simulink library "simeventsserver1"  (Simulink 7.5)
settings: Solver=ode45  SolverMode=SingleTasking  StartTime=0.0  StopTime=10.0  RelTol=1e-3
undefined symbols (not defined in the file or in its folder): des_support, gcbh
settings Model: Creator=mclune  LastModifiedBy=ywu  ExtModeAutoUpdateStatusClock=off

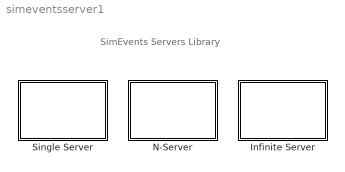
== system simeventsserver1 ==
  note: SimEvents Servers Library
  Infinite Server : Subsystem  Priority=1  LoadFcn=des_support('desLoadFcn',gcbh)  StartFcn=des_support('desStartFcn',gcbh)  StopFcn=des_support('desStopFcn',gcbh)  mask(Infinite Server){ServiceTimeFrom=Dialog, ServiceTime=1, AttributeName=ServiceTime, PriorityServiceCompletion=500, EnableTOPort=off, StatNumberDeparted=Off, StatNumberInBlock=Off, StatPendingEntity=Off, StatNumberPending=Off, StatAverageWait=Off, StatNumberTimedout=Off}
      mask prompts: ServiceTimeFrom "Service time from:"; ServiceTime "Service time:"; AttributeName "Attribute name:"; PriorityServiceCompletion "Service completion event priority:"; EnableTOPort "Enable TO port for timed-out entities:"; StatNumberDeparted "Number of entities departed, #d:"; StatNumberInBlock "Number of entities in block, #n:"; StatPendingEntity "Pending entity present in block, pe:"; StatNumberPending "Number of  pending entities, #pe:"; StatAverageWait "Average wait, w:"; StatNumberTimedout "Number of entities timed-out, #to:"
      mask help:
      | Delay any number of entities for a period of time and then attempt to output through the OUT port. If the OUT port is blocked then the entities stay in this block until the port becomes unblocked. You can specify the delay time via a parameter, attribute, or signal.
      | This block is an infinite server so the IN port is always available.
      mask init:
      | des_delaymask(gcb, 'init','apply')
      settings: CopyFcn=des_support('desCopyFcn',gcbh)  DeleteFcn=des_support('desDeleteFcn',gcbh)  UndoDeleteFcn=des_support('desUndoDeleteFcn',gcbh)  ModelCloseFcn=des_support('desModelCloseFcn',gcbh)  PreSaveFcn=des_support('desPreSaveFcn',gcbh)  PostSaveFcn=des_support('desPostSaveFcn',gcbh)  NameChangeFcn=des_support('desNameChangeFcn',gcbh)  CloseFcn=des_support('desCloseFcn',gcbh)  ErrorFcn=des_error_redirect
      mask Help: helpview(simeventsbhelp)
      mask StyleString: popup(Dialog|Signal port t|Attribute),edit,edit,edit,checkbox,popup(Off|On|Upon stop or pause),popup(Off|On|Upon stop or pause),popup(Off|On),popup(Off|On|Upon stop or pause),popup(Off|On|Upon stop or pause),popup(Off|On|Upon stop or pause)
      mask CallbackString: des_delaymask(gcb,'cbServiceTimeFrom','noapply');||||des_delaymask(gcb,'cbEnableTOPort','noapply');|des_delaymask(gcb,'cbStatNumberDeparted','noapply');|des_delaymask(gcb,'cbStatNumberInBlock','noapply');|des_delaymask(gcb,'cbStatPendingEntity','noapply');|des_delaymask(gcb,'cbStatNumberPending','noapply');|des_delaymask(gcb,'cbStatAverageWait','noapply');|des_delaymask(gcb,'cbStatNumberTimedout','noapply');
      mask TabNameString: Infinite Server,Infinite Server,Infinite Server,Infinite Server,Timeout,Statistics,Statistics,Statistics,Statistics,Statistics,Statistics
      mask Display:
      | image(des_iconLoad('serverInf.jpg'),'center');
      | port_label('LConn',1,'IN');
      | port_label('RConn',1,'OUT');
  N-Server : Subsystem  Priority=1  LoadFcn=des_support('desLoadFcn',gcbh)  StartFcn=des_support('desStartFcn',gcbh)  StopFcn=des_support('desStopFcn',gcbh)  mask(N-Server){NumberOfServers=5, ServiceTimeFrom=Dialog, ServiceTime=1, AttributeName=ServiceTime, PriorityServiceCompletion=500, EnableTOPort=off, StatNumberDeparted=Off, StatNumberInBlock=Off, StatPendingEntity=Off, StatNumberPending=Off, StatAverageWait=Off, StatUtilization=Off, StatNumberTimedout=Off}
      mask prompts: NumberOfServers "Number of servers:"; ServiceTimeFrom "Service time from:"; ServiceTime "Service time:"; AttributeName "Attribute name:"; PriorityServiceCompletion "Service completion event priority:"; EnableTOPort "Enable TO port for timed-out entities"; StatNumberDeparted "Number of entities departed, #d:"; StatNumberInBlock "Number of entities in block, #n:"; StatPendingEntity "Pending entity present in block, pe:"; StatNumberPending "Number of pending entities, #pe:"; StatAverageWait "Average wait, w:"; StatUtilization "Utilization, util:"; StatNumberTimedout "Number of entities timed-out, #to:"
      mask help:
      | Serve up to N entities independently for a period of time and then attempt to output each entity through the OUT port. If the OUT port is blocked then the pending entity stays in this block until the port becomes unblocked. You can specify the service time, which is the duration of service, via a parameter, attribute, or signal.
      |
      | The IN port is unavailable whenever the number of entities stored is N.
      mask init:
      | des_nservermask(gcb, 'init','apply')
      settings: CopyFcn=des_support('desCopyFcn',gcbh)  DeleteFcn=des_support('desDeleteFcn',gcbh)  UndoDeleteFcn=des_support('desUndoDeleteFcn',gcbh)  ModelCloseFcn=des_support('desModelCloseFcn',gcbh)  PreSaveFcn=des_support('desPreSaveFcn',gcbh)  PostSaveFcn=des_support('desPostSaveFcn',gcbh)  NameChangeFcn=des_support('desNameChangeFcn',gcbh)  CloseFcn=des_support('desCloseFcn',gcbh)  ErrorFcn=des_error_redirect
      mask Help: helpview(simeventsbhelp)
      mask StyleString: edit,popup(Dialog|Signal port t|Attribute),edit,edit,edit,checkbox,popup(Off|On|Upon stop or pause),popup(Off|On|Upon stop or pause),popup(Off|On),popup(Off|On|Upon stop or pause),popup(Off|On|Upon stop or pause),popup(Off|On|Upon stop or pause),popup(Off|On|Upon stop or pause)
      mask CallbackString: |des_nservermask(gcb,'cbServiceTimeFrom','noapply');||||des_nservermask(gcb,'cbEnableTOPort','noapply');|des_nservermask(gcb,'cbStatNumberDeparted','noapply');|des_nservermask(gcb,'cbStatNumberInBlock','noapply');|des_nservermask(gcb,'cbStatPendingEntity','noapply');|des_nservermask(gcb,'cbStatNumberPending','noapply');|des_nservermask(gcb,'cbStatAverageWait','noapply');|des_nservermask(gcb,'cbStatUtilization','noapply');|des_nservermask(gcb,'cbStatNumberTimedout','noapply');
      mask TabNameString: N-Server,N-Server,N-Server,N-Server,N-Server,Timeout,Statistics,Statistics,Statistics,Statistics,Statistics,Statistics,Statistics
      mask Display:
      | image(des_iconLoad('serverN.jpg'),'center');
      | port_label('LConn',1,'IN');
      | port_label('RConn',1,'OUT');
  Single Server : Subsystem  Priority=1  LoadFcn=des_support('desLoadFcn',gcbh)  StartFcn=des_support('desStartFcn',gcbh)  StopFcn=des_support('desStopFcn',gcbh)  mask(Single Server){ServiceTimeFrom=Dialog, ServiceTime=1, AttributeName=ServiceTime, PriorityServiceCompletion=500, PermitPreemption=off, SortingAttributeName=PriorityAttributeName, SortingDirection=Ascending, WriteToAttribute=off, ResidualAttributeName=ResidualServiceTime, CreateAttribute=on, EnableTOPort=off, StatNumberDeparted=Off, StatNumberInBlock=Off, StatNumberPreempted=Off, StatPendingEntity=Off, StatAverageWait=Off, StatUtilization=Off, StatNumberTimedout=Off}
      mask prompts: ServiceTimeFrom "Service time from:"; ServiceTime "Service time:"; AttributeName "Attribute name:"; PriorityServiceCompletion "Service completion event priority:"; PermitPreemption "Permit preemption based on attribute"; SortingAttributeName "Sorting attribute name:"; SortingDirection "Sorting direction:"; WriteToAttribute "Write residual service time to attribute"; ResidualAttributeName "Residual service time attribute name:"; CreateAttribute "Create attribute if not present"; EnableTOPort "Enable TO port for timed-out entities"; StatNumberDeparted "Number of entities departed, #d:"; StatNumberInBlock "Number of entities in block, #n:"; StatNumberPreempted "Number of entities preempted, #p:"; StatPendingEntity "Pending entity present in block, pe:"; StatAverageWait "Average wait, w:"; StatUtilization "Utilization, util:"; StatNumberTimedout "Number of entities timed-out, #to:"
      mask help:
      | Serve one entity for a period of time and then attempt to output the entity through the OUT port. If the OUT port is blocked then the entity stays in this block until the port becomes unblocked. You can specify the service time, which is the duration of service, via a parameter, attribute, or signal.
      |
      | When the block permits preemption, an entity in the server can depart early via the P port. Preemption occurs only if attributes of the current entity and the entity attempting to arrive satisfy specified criteria.
      |
      | When the block does not permit preemption, the IN port is unavailable whenever this block stores an entity.
      mask init:
      | des_basicservermask(gcb, 'init','apply')
      settings: CopyFcn=des_support('desCopyFcn',gcbh)  DeleteFcn=des_support('desDeleteFcn',gcbh)  UndoDeleteFcn=des_support('desUndoDeleteFcn',gcbh)  ModelCloseFcn=des_support('desModelCloseFcn',gcbh)  PreSaveFcn=des_support('desPreSaveFcn',gcbh)  PostSaveFcn=des_support('desPostSaveFcn',gcbh)  NameChangeFcn=des_support('desNameChangeFcn',gcbh)  CloseFcn=des_support('desCloseFcn',gcbh)  ErrorFcn=des_error_redirect
      mask Help: helpview(simeventsbhelp)
      mask StyleString: popup(Dialog|Signal port t|Attribute),edit,edit,edit,checkbox,edit,popup(Ascending|Descending),checkbox,edit,checkbox,checkbox,popup(Off|On|Upon stop or pause),popup(Off|On|Upon stop or pause),popup(Off|On|Upon stop or pause),popup(Off|On),popup(Off|On|Upon stop or pause),popup(Off|On|Upon stop or pause),popup(Off|On|Upon stop or pause)
      mask CallbackString: des_basicservermask(gcb,'cbServiceTimeFrom','noapply');|des_basicservermask(gcb,'cbServiceTime','noapply');|des_basicservermask(gcb,'cbAttributeName','noapply');||des_basicservermask(gcb,'cbPermitPreemption','noapply');|||des_basicservermask(gcb,'cbResidualAttributeName','noapply');|||des_basicservermask(gcb,'cbEnableTOPort','noapply');|des_basicservermask(gcb,'cbStatNumberDeparted','noapply');|des_basicservermask(gcb,'cbStatNumberInBlock','noapply');|des_basicservermask(gcb,'cbStatNumberPreempted','noapply');|des_basicservermask(gcb,'cbStatPendingEntity','noapply');|des_basicservermask(gcb,'cbStatAverageWait','noapply');|des_basicservermask(gcb,'cbStatUtilization','noapply');|des_basicservermask(gcb,'cbStatNumberTimedout','noapply');
      mask TabNameString: Single Server,Single Server,Single Server,Single Server,Preemption,Preemption,Preemption,Preemption,Preemption,Preemption,Timeout,Statistics,Statistics,Statistics,Statistics,Statistics,Statistics,Statistics
      mask Display:
      | image(des_iconLoad('serverSingle.jpg'),'center');
      | port_label('LConn',1,'IN');
      | port_label('RConn',1,'OUT');

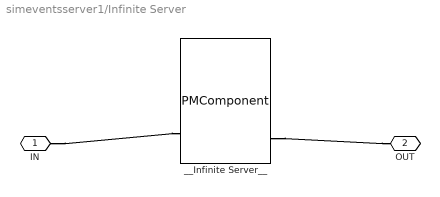
== system simeventsserver1/Infinite Server ==
  __Infinite Server__ : PMComponent  PhysicalDomain=simevents  SubClassName=DES_DELAY  LeftPortType=desPortIn  RightPortType=desPortOut  LConnTagsString=DI|DI  RConnTagsString=DO|DO|DO|DO|DO|DO|DO|DO
      mask Display:
      | port_label('LConn',1,'t');
      | port_label('LConn',2,'IN');
      | port_label('RConn',1,'#d');
      | port_label('RConn',2,'#n');
      | port_label('RConn',3,'pe');
      | port_label('RConn',4,'#pe');
      | port_label('RConn',5,'w');
      | port_label('RConn',6,'#to');
      | port_label('RConn',7,'OUT');
      | port_label('RConn',8,'TO');
  IN : PMIOPort  Port=1  Side=Left
  OUT : PMIOPort  Port=2  Side=Right
  connections:
  IN/RConn1 -- __Infinite Server__/LConn2
  __Infinite Server__/RConn7 -- OUT/RConn1

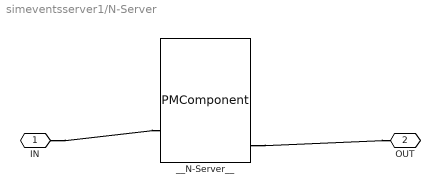
== system simeventsserver1/N-Server ==
  __N-Server__ : PMComponent  PhysicalDomain=simevents  SubClassName=DES_NSERVER  LeftPortType=desPortIn  RightPortType=desPortOut  LConnTagsString=DI|DI  RConnTagsString=DO|DO|DO|DO|DO|DO|DO|DO|DO
      mask Display:
      | port_label('LConn',1,'t');
      | port_label('LConn',2,'IN');
      | port_label('RConn',1,'#d');
      | port_label('RConn',2,'#n');
      | port_label('RConn',3,'pe');
      | port_label('RConn',4,'#pe');
      | port_label('RConn',5,'w');
      | port_label('RConn',6,'util');
      | port_label('RConn',7,'#to');
      | port_label('RConn',8,'OUT');
      | port_label('RConn',9,'TO');
  IN : PMIOPort  Port=1  Side=Left
  OUT : PMIOPort  Port=2  Side=Right
  connections:
  IN/RConn1 -- __N-Server__/LConn2
  __N-Server__/RConn8 -- OUT/RConn1

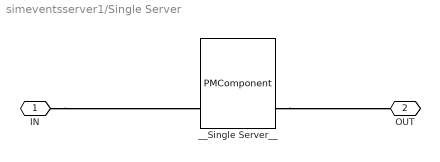
== system simeventsserver1/Single Server ==
  __Single Server__ : PMComponent  PhysicalDomain=simevents  SubClassName=DES_BASICSERVER  LeftPortType=desPortIn  RightPortType=desPortOut  LConnTagsString=DI|DI  RConnTagsString=DO|DO|DO|DO|DO|DO|DO|DO|DO|DO
      mask Display:
      | port_label('LConn',1,'t');
      | port_label('LConn',2,'IN');
      | port_label('RConn',1,'#d');
      | port_label('RConn',2,'#n');
      | port_label('RConn',3,'#p');
      | port_label('RConn',4,'pe');
      | port_label('RConn',5,'w');
      | port_label('RConn',6,'util');
      | port_label('RConn',7,'#to');
      | port_label('RConn',8,'OUT');
      | port_label('RConn',9,'P');
      | port_label('RConn',10,'TO');
  IN : PMIOPort  Port=1  Side=Left
  OUT : PMIOPort  Port=2  Side=Right
  connections:
  IN/RConn1 -- __Single Server__/LConn2
  __Single Server__/RConn8 -- OUT/RConn1
